simulink model "holiday7"  (R2019a)
settings: Solver=VariableStepAuto  StartTime=0.0  StopTime=10.0  RelTol=1e-3
undefined symbols (not defined in the file or in its folder): aditya
settings Model: Creator=Aditya  LastModifiedBy=Aditya

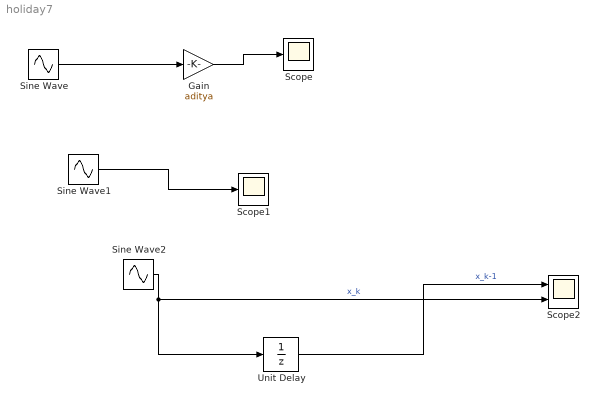
== system holiday7 ==
  Gain : Gain  Gain=aditya
  Scope : Scope
  Scope1 : Scope
  Scope2 : Scope  NumInputPorts=2
  Sine Wave : Sin  SampleTime=0
  Sine Wave1 : Sin  Amplitude=aditya  SampleTime=0
  Sine Wave2 : Sin  Amplitude=aditya  SampleTime=0.25
  Unit Delay : UnitDelay  SampleTime=-1  HasFrameUpgradeWarning=on
  wires:
  Sine Wave/1 -> Gain/1
  Gain/1 -> Scope/1
  Sine Wave1/1 -> Scope1/1
  Sine Wave2/1 -> Unit Delay/1, Scope2/2  "x_k"
  Unit Delay/1 -> Scope2/1  "x_k-1"
